simulink model "hexa_tilted_PID"  (R2022b)
settings: Solver=ode4  StartTime=0.0  StopTime=tf  FixedStep=0.01  RelTol=1e-3
model workspace (MAT data in the model file):
  tf = Simulink.Parameter
  tf.Value = 60
  tf.DataType = 'auto'
  tf.Complexity = 'real'
  tf.Dimensions = [1 1]
  tray1 = [0  2  2  -2  0  0; 0  -2  -2  2  0  0; 0  5  2.5  5  2.5  0; 0  0  0  0  0  0; 0  0  0  0  0  0; 0  0  1.57  0  0  0]
  tray2 = [0  2  2  -2  0  0; 0  -2  -2  2  0  0; 0  5  2.5  5  2.5  0; 0  0  0  0  0  0; 0  0  0  0  0  0; 0  0  0  0  0  0]
libraries: robotcorelib x1
settings Model: Creator=adan  LastModifiedBy=Adan Daniel

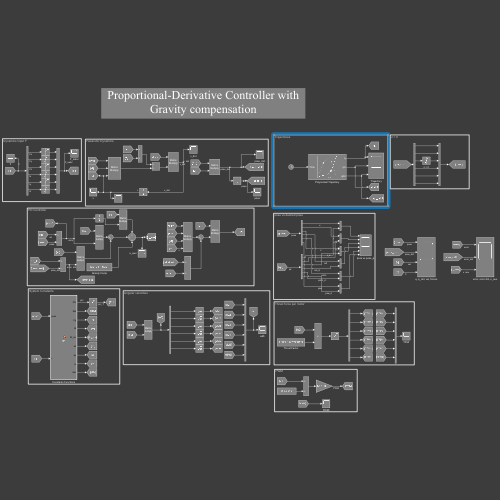
[thumbnail: Simulink's stored preview of the top-level diagram]
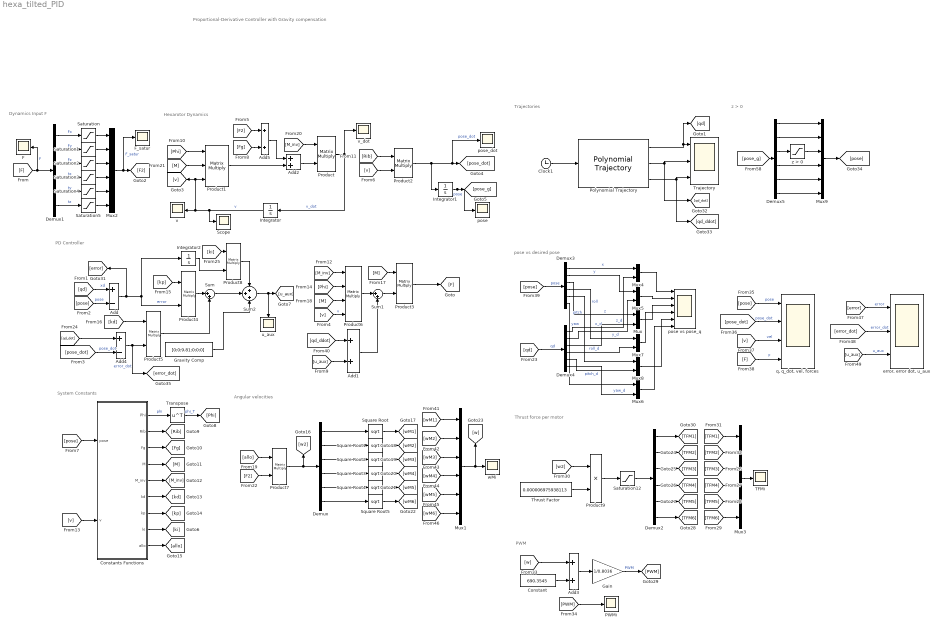
== system hexa_tilted_PID ==
  note: Trajectories
  note: PWM
  note: System Constants
  note: Angular velocities
  note: Thrust force per motor
  note: PD Controller
  note: Hexarotor Dynamics
  note: Dynamics Input F
  note: Proportional-Derivative Controller with Gravity compensation
  note: z > 0
  note: pose vs desired pose
  Add : Sum  Inputs=+-
  Add{1..3,5} (4 alike) : Sum
  Add4 : Sum  Inputs=+-
  Clock1 : Clock
  Constant : Constant  Value=690.3545
  Constants Functions : MATLAB Function  TreatAsAtomicUnit=on
  Demux{,1..5} (6 alike) : Demux  Outputs=6
  F : Scope
  F_satur : Scope
  Gain : Gain  Gain=1/0.8036
  Gravity Comp : Constant  Value=[0;0;9.81;0;0;0]
  Integrator : Integrator  InitialCondition=[0; 0; 0; 0; 0; 0]
  Integrator1 : Integrator  InitialCondition=[0; 0; 0; 0; 0; 0]
  Integrator2 : Integrator
  Mux{,4..8} (6 alike) : Mux  Inputs=2
  Mux{1..3,9} (4 alike) : Mux  Inputs=6
  PWMi : Scope
  Polynomial Trajectory : robotcorelib/Polynomial Trajectory  WaypointSource=Internal  Waypoints=tray1  TimePoints=[ 0, 5, 20, 28, 54, tf ]  TimeInterval=[ 1, 4 ]  Method=Cubic Polynomial  ParameterSource=Internal  VelocityBoundaryCondition=zeros( 6, 6 )  AccelerationBoundaryCondition=zeros( 2, 5 )  SimulateUsing=Interpreted execution
  Product{,2..5,7..8} (7 alike) : Product  Multiplication=Matrix(*)
  Product1 : Product  Inputs=3  Multiplication=Matrix(*)
  Product6 : Product  Inputs=4  Multiplication=Matrix(*)
  Product9 : Product
  Saturation : Saturate  UpperLimit=6  LowerLimit=-6
  Saturation1 : Saturate  UpperLimit=6  LowerLimit=-6
  Saturation12 : Saturate  UpperLimit=818608.7529  LowerLimit=0
  Saturation2 : Saturate  UpperLimit=5.8*6  LowerLimit=0
  Saturation3 : Saturate
  Saturation4 : Saturate
  Saturation5 : Saturate
  Scope : Scope
  Square Root{,1..5} (6 alike) : Sqrt
  Sum : Sum  Inputs=|++
  Sum1 : Sum  Inputs=|++
  Sum2 : Sum  Inputs=+++
  TFMi : Scope
  Thrust Factor : Constant  Value=0.000006975938113
  Trajectory : Scope  NumInputPorts=3
  Transpose : Math  Operator=transpose
  "error, error dot, u_aux" : Scope  NumInputPorts=3
  pose : Scope
  pose vs pose_q : Scope  NumInputPorts=6
  pose_dot : Scope
  "q, q_dot, vel, forces" : Scope  NumInputPorts=4
  u_aux : Scope
  v : Scope
  v_dot : Scope
  wMi : Scope
  z > 0 : Saturate  UpperLimit=100  LowerLimit=0
  wires:
  Saturation/1 -> Mux2/1
  Saturation1/1 -> Mux2/2
  Saturation4/1 -> Mux2/5
  Saturation3/1 -> Mux2/4
  Demux1/6 -> Saturation5/1  "tz"
  Demux1/3 -> Saturation2/1  "Fz"
  [F] -> F/1, Demux1/1  "F"
  Saturation5/1 -> Mux2/6
  Demux1/2 -> Saturation1/1  "Fy"
  Demux1/1 -> Saturation/1  "Fx"
  Demux1/5 -> Saturation4/1  "ty"
  Demux1/4 -> Saturation3/1  "tx"
  Saturation2/1 -> Mux2/3
  Mux2/1 -> F_satur/1, [F2]  "F_satur"
  [M] -> Product1/2
  [v] -> Product2/2
  [M_inv] -> Product/1
  Add2/1 -> Product/2
  Product/1 -> v_dot/1, Integrator/1  "v_dot"
  [Rib] -> Product2/1
  Product2/1 -> pose_dot/1, [pose_dot], Integrator1/1  "pose_dot"
  [Phi] -> Product1/1
  Product1/1 -> Add2/2
  Integrator1/1 -> pose/1, [pose_g]  "pose"
  Integrator/1 -> Scope/1, v/1, [v], Product1/3  "v"
  [Fg] -> Add5/2
  Add5/1 -> Add2/1
  [pose_dot] -> Add4/2  "pose_dot"
  [qd_dot] -> Add4/1
  [Phi] -> Product6/2
  Add4/1 -> [error_dot], Product5/2  "error_dot"
  [qd_ddot] -> Add1/1
  [qd] -> Add/1  "xd"
  [kp] -> Product4/1
  [v] -> Product6/4  "v"
  [kd] -> Product5/1
  Product4/1 -> Sum/1
  [pose] -> Add/2  "pose"
  [M_inv] -> Product6/1
  [M] -> Product6/3
  Add/1 -> [error], Product4/2, Integrator2/1  "error"
  Product5/1 -> Sum/2
  [u_aux] -> Add1/2
  Sum2/1 -> u_aux/1, [u_aux]
  [F2] -> Add5/1
  [ki] -> Product8/1
  Integrator2/1 -> Product8/2
  Gravity Comp/1 -> Sum2/3
  Sum/1 -> Sum2/2
  Product8/1 -> Sum2/1
  Add1/1 -> Sum1/2
  [TFM6] -> Mux3/6
  Demux2/2 -> [TFM2]
  [TFM3] -> Mux3/3
  Demux2/6 -> [TFM6]
  [TFM5] -> Mux3/5
  Saturation12/1 -> Demux2/1
  [TFM2] -> Mux3/2
  [TFM1] -> Mux3/1
  Demux2/5 -> [TFM5]
  Demux2/4 -> [TFM4]
  Product9/1 -> Saturation12/1
  Demux2/1 -> [TFM1]
  Thrust Factor/1 -> Product9/2
  Demux2/3 -> [TFM3]
  [w2] -> Product9/1
  [TFM4] -> Mux3/4
  [wM1] -> Mux1/1
  Square Root/1 -> [wM1]
  [wM5] -> Mux1/5
  Square Root5/1 -> [wM6]
  Square Root3/1 -> [wM4]
  [F2] -> Product7/2
  [allo] -> Product7/1
  [wM2] -> Mux1/2
  Demux/6 -> Square Root5/1
  Demux/5 -> Square Root4/1
  Square Root1/1 -> [wM2]
  [wM3] -> Mux1/3
  Square Root2/1 -> [wM3]
  Demux/4 -> Square Root3/1
  Demux/2 -> Square Root1/1
  Demux/3 -> Square Root2/1
  Square Root4/1 -> [wM5]
  Product7/1 -> [w2], Demux/1
  Demux/1 -> Square Root/1
  [wM4] -> Mux1/4
  Mux1/1 -> [w], wMi/1
  [wM6] -> Mux1/6
  Constants Functions/2(Rib) -> [Rib]
  [pose] -> Constants Functions/1(pose)
  Constants Functions/1(Phi) -> Transpose/1  "phi"
  Constants Functions/4(M) -> [M]
  Constants Functions/7(kp) -> [kp]
  Constants Functions/5(M_inv) -> [M_inv]
  Constants Functions/8(ki) -> [ki]
  Constants Functions/9(allo) -> [allo]
  Constants Functions/3(Fg) -> [Fg]
  Transpose/1 -> [Phi]  "phi_T"
  Constants Functions/6(kd) -> [kd]
  [v] -> Constants Functions/2(v)
  Mux3/1 -> TFMi/1
  Constant/1 -> Add3/2
  [PWM] -> PWMi/1
  [w] -> Add3/1
  Gain/1 -> [PWM]  "PWM"
  Add3/1 -> Gain/1
  Clock1/1 -> Polynomial Trajectory/1
  Polynomial Trajectory/2 -> Trajectory/2, [qd_dot]
  Polynomial Trajectory/3 -> Trajectory/3, [qd_ddot]
  Polynomial Trajectory/1 -> [qd], Trajectory/1
  [pose_dot] -> "q, q_dot, vel, forces"/2  "pose_dot"
  [pose] -> "q, q_dot, vel, forces"/1  "pose"
  [F] -> "q, q_dot, vel, forces"/4  "F"
  [v] -> "q, q_dot, vel, forces"/3  "vel"
  Product6/1 -> Sum1/1
  Sum1/1 -> Product3/2
  [M] -> Product3/1
  Product3/1 -> [F]
  Demux5/1 -> Mux9/1
  Demux5/4 -> Mux9/4
  Demux5/3 -> z > 0/1
  Demux5/2 -> Mux9/2
  z > 0/1 -> Mux9/3
  [pose_g] -> Demux5/1
  Demux5/6 -> Mux9/6
  Mux9/1 -> [pose]
  Demux5/5 -> Mux9/5
  Demux3/5 -> Mux8/1  "pitch"
  Demux4/4 -> Mux7/2  "roll_d"
  Demux3/2 -> Mux5/1  "y"
  Mux5/1 -> pose vs pose_q/2
  Demux3/3 -> Mux/1  "z"
  [qd] -> Demux4/1  "qd"
  Mux8/1 -> pose vs pose_q/5
  Mux7/1 -> pose vs pose_q/4
  Mux4/1 -> pose vs pose_q/1
  Demux4/6 -> Mux6/2  "yaw_d"
  Demux4/1 -> Mux4/2  "x_d"
  Demux3/1 -> Mux4/1  "x"
  Demux3/4 -> Mux7/1  "roll"
  Mux6/1 -> pose vs pose_q/6
  [pose] -> Demux3/1  "pose"
  Mux/1 -> pose vs pose_q/3
  Demux4/5 -> Mux8/2  "pitch_d"
  Demux4/3 -> Mux/2  "z_d"
  Demux3/6 -> Mux6/1  "yaw"
  Demux4/2 -> Mux5/2  "y_d"
  [error_dot] -> "error, error dot, u_aux"/2  "error_dot"
  [error] -> "error, error dot, u_aux"/1  "error"
  [u_aux] -> "error, error dot, u_aux"/3  "u_aux"

== matlab function hexa_tilted_PID/Constants Functions ==
  data: Phi output; Rib output; Fg output; pose input; M output; M_inv output; kd output; kp output; ki output; allo output; v input
function [Phi, Rib, Fg, M, M_inv, kd, kp, ki, allo] = fcn(pose, v)

%% system constants
pi = 3.141592;
m = 2.0; %5 mass 2.2 kg
l = 0.25; % length m
g = 9.81; % gravity m/s²
Jxx =  24778420.82/(1000*1000000); % kg m²
Jyy = 42217933.96/(1000*1000000); % kg m²
Jzz = 23948304.24/(1000*1000000); % kg m²
kT = 0.000006975938113;
kQ = 0.000118290418538;

%% Phi matrix calculation
uu = v(1);
vv = v(2);
ww = v(3);
pp = v(4);
qq = v(5);
rr = v(6);


Phi = [0, -rr, qq, 0, -ww, vv;
        rr, 0, -pp , ww, 0, -uu;
        -qq, pp, 0,  -vv, uu, 0;
        0, 0, 0, 0, -rr, qq; 
        0, 0, 0, rr, 0, -pp;
        0, 0, 0, -qq, pp, 0];

%% Rib matrix calculation

roll = pose(4);
pitch = pose(5);
yaw = pose(6);

Rib = [cos(yaw)*cos(pitch), -cos(roll)*sin(yaw) + cos(yaw)*sin(roll)*sin(pitch), sin(roll)*sin(yaw) + cos(roll)*cos(yaw)*sin(pitch), 0, 0, 0;
       cos(pitch)*sin(yaw), cos(roll)*cos(yaw) + sin(yaw)*sin(pitch)*sin(roll), -cos(yaw)*sin(roll) + sin(yaw)*sin(pitch)*cos(roll), 0, 0, 0;
       -sin(pitch), cos(pitch)*sin(roll), cos(pitch)*cos(roll), 0, 0, 0;
       0, 0, 0, 1, sin(roll)*tan(pitch), cos(roll)*tan(pitch);
       0, 0, 0, 0, cos(roll), -sin(roll);
       0, 0, 0, 0, sin(roll)/cos(pitch), cos(roll)/cos(pitch)];

%% Fg matrix calculation

Fg = [m*g*sin(pitch);
      -m*g*cos(pitch)*sin(roll);
      -m*g*cos(pitch)*cos(roll);
      0;
      0;
      0];

%% Constantes proporcionales
% más grande más rapido subo 

kp_x = 6;
kp_y = 4.5;
kp_z = 2;
kp_roll = 20;
kp_pitch = 20;
kp_yaw = 2;

%% Constantes derivativas
% atenuar oscilación 
kd_x = 5;
kd_y = 4.5;
kd_z = 7;
kd_roll = 5;
kd_pitch = 3;
kd_yaw = 3;

%% Constantes integrales

ki_x = 0;
ki_y = 0;
ki_z = 0;
ki_roll = 0;
ki_pitch = 0;
ki_yaw = 0;

varphi = pi/9;

kp = [kp_x, 0, 0, 0, 0, 0;
      0, kp_y, 0, 0, 0, 0;
      0, 0, kp_z, 0, 0, 0;
      0, 0, 0, kp_roll, 0, 0;
      0, 0, 0, 0, kp_pitch, 0;
      0, 0, 0, 0, 0, kp_yaw];

kd = [kd_x, 0, 0, 0, 0, 0;
      0, kd_y, 0, 0, 0, 0;
      0, 0, kd_z, 0, 0, 0;
      0, 0, 0, kd_roll, 0, 0;
      0, 0, 0, 0, kd_pitch, 0;
      0, 0, 0, 0, 0, kd_yaw];

ki = [ki_x, 0, 0, 0, 0, 0;
      0, ki_y, 0, 0, 0, 0;
      0, 0, ki_z, 0, 0, 0;
      0, 0, 0, ki_roll, 0, 0;
      0, 0, 0, 0, ki_pitch, 0;
      0, 0, 0, 0, 0, ki_yaw];

M = [m, 0, 0, 0, 0, 0;
    0, m, 0, 0, 0, 0;
    0, 0, m, 0, 0, 0;
    0, 0, 0, Jxx, 0, 0;
    0, 0, 0, 0, Jyy, 0;
    0, 0, 0, 0, 0, Jzz];

M_inv = inv(M);

alpha = [pi/6; -pi/6; -pi/2; -5*pi/6; 5*pi/6; pi/2];

%% tilted rotors matrix allocation

m11 = -kT*cos(alpha(1))*sin(varphi);
m21 = kT*sin(alpha(1))*sin(varphi);
m31 = kT*cos(varphi);
m41 = cos(alpha(1))*(l*kT*cos(varphi) - kQ*sin(varphi));
m51 = sin(alpha(1))*(-l*kT*cos(varphi) + kQ*sin(varphi));
m61 = l*kT*sin(varphi) + kQ*cos(varphi);

m12 = kT*cos(alpha(2))*sin(varphi);
m22 = -kT*sin(alpha(2))*sin(varphi);
m32 = m31;
m42 = cos(alpha(2))*(l*kT*cos(varphi) - kQ*sin(varphi));
m52 = sin(alpha(2))*(-l*kT*cos(varphi) + kQ*sin(varphi));
m62 = -l*kT*sin(varphi) - kQ*cos(varphi);

m13 = kT*cos(alpha(3))*sin(varphi);
m23 = kT*sin(alpha(3))*sin(varphi);
m33 = m31;
m43 = cos(alpha(3))*(l*kT*cos(varphi) + kQ*sin(varphi));
m53 = sin(alpha(3))*(-l*kT*cos(varphi) + kQ*sin(varphi));
m63 = l*kT*sin(varphi) + kQ*cos(varphi);

m14 = kT*cos(alpha(4))*sin(varphi);
m24 = -kT*sin(alpha(4))*sin(varphi);
m34 = m31;
m44 = cos(alpha(4))*(l*kT*cos(varphi) - kQ*sin(varphi));
m54 = sin(alpha(4))*(-l*kT*cos(varphi) + kQ*sin(varphi));
m64 = -l*kT*sin(varphi) - kQ*cos(varphi);

m15 = -kT*cos(alpha(5))*sin(varphi);
m25 = kT*sin(alpha(5))*sin(varphi);
m35 = m31;
m45 = cos(alpha(5))*(l*kT*cos(varphi) - kQ*sin(varphi));
m55 = sin(alpha(5))*(-l*kT*cos(varphi) + kQ*sin(varphi));
m65 = l*kT*sin(varphi) + kQ*cos(varphi);

m16 = kT*cos(alpha(6))*sin(varphi);
m26 = -kT*sin(alpha(6))*sin(varphi);
m36 = m31;
m46 = cos(alpha(6))*(l*kT*cos(varphi) + kQ*sin(varphi));
m56 = sin(alpha(6))*(-l*kT*cos(varphi) + kQ*sin(varphi));
m66 = -l*kT*sin(varphi) - kQ*cos(varphi);

allo = [m11, m12, m13, m14, m15, m16;
        m21, m22, m23, m24, m25, m26;
        m31, m32, m33, m34, m35, m36;
        m41, m42, m43, m44, m45, m46;
        m51, m52, m53, m54, m55, m56;
        m61, m62, m63, m64, m65, m66];

allo = inv(allo);

Ref = 0;
